simulink library "CockpitDisplayLib"  (R2013b)
settings: Solver=ode45  StartTime=0.0  StopTime=10.0  RelTol=1e-3
undefined symbols (not defined in the file): Ts
libraries: dspadpt3 x3, sf_aircraft_screen_library x1, LandingGearModeLib x1
(part 2 of 2)

== stateflow chart CockpitDisplayLib/Warnings/ComponentModes.RPM ==
  state Normal
    entry: RPMProblem = 0;
  state EngineFailure
    entry:
    RPMProblem = 1;
  state EngineOverSpeed
    entry:
    RPMProblem = 2;
  (default) -> Normal
  Normal -> EngineFailure [order 1] : [funcNormalToEngFailure]
  Normal -> EngineOverSpeed [order 2] : [FlightMode == 1 ...
      | && EngNFuel.RPM >10000]
  EngineFailure -> Normal : [funcEngFailureToNormal]
  EngineOverSpeed -> Normal : [~(FlightMode == 1 ...
      | && EngNFuel.RPM >10000)]
  data: y function_output boolean size=1; y function_output boolean size=1; EngNFuel input Bus: EngineFuel_Bus; RPMProblem output double size=1; FlightMode data_store_memory size=1
  function y = funcEngFailureToNormal:
    | function y = funcEngFailureToNormal
    | 
    | aVarTruthTableCondition_1 = false;
    | aVarTruthTableCondition_2 = false;
    | aVarTruthTableCondition_3 = false;
    | aVarTruthTableCondition_4 = false;
    | 
    | 
    | 
    | aVarTruthTableCondition_1 = logical(FlightMode == 1);
    | 
    | 
    | aVarTruthTableCondition_2 = logical(FlightMode == 2);
    | 
    | 
    | aVarTruthTableCondition_3 = logical(EngNFuel.RPM < 700);
    | 
    | 
    | aVarTruthTableCondition_4 = logical(EngNFuel.RPM < 1500);
    | 
    | if (aVarTruthTableCondition_1 && aVarTruthTableCondition_3)
    |     aFcnTruthTableAction_2();
    | elseif (aVarTruthTableCondition_2 && aVarTruthTableCondition_4)
    |     aFcnTruthTableAction_2();
    | else % Default
    |     aFcnTruthTableAction_1();
    | end
    | 
    | function aFcnTruthTableAction_1()
    | 
    | 
    | y = true;
    | 
    | function aFcnTruthTableAction_2()
    | 
    | 
    | y = false;
  function y = funcNormalToEngFailure:
    | function y = funcNormalToEngFailure
    | 
    | aVarTruthTableCondition_1 = false;
    | aVarTruthTableCondition_2 = false;
    | aVarTruthTableCondition_3 = false;
    | aVarTruthTableCondition_4 = false;
    | 
    | 
    | % Is the aircraft in the PushbackAndTaxi phase
    | 
    | aVarTruthTableCondition_1 = logical(FlightMode == 1);
    | 
    | % Is the aircraft in the TakeoffCruiseDescent phase
    | 
    | aVarTruthTableCondition_2 = logical(FlightMode == 2);
    | 
    | % Lower Threshold for engine speed in PushbackAndTaxi
    | 
    | aVarTruthTableCondition_3 = logical(EngNFuel.RPM < 650);
    | 
    | % Lower Threshold for engine speed in TakeoffCruiseDescent
    | 
    | aVarTruthTableCondition_4 = logical(EngNFuel.RPM < 1500);
    | 
    | if (aVarTruthTableCondition_1 && aVarTruthTableCondition_3)
    |     aFcnTruthTableAction_1();
    | elseif (aVarTruthTableCondition_2 && aVarTruthTableCondition_4)
    |     aFcnTruthTableAction_1();
    | else % Default
    |     aFcnTruthTableAction_2();
    | end
    | 
    | function aFcnTruthTableAction_1()
    | 
    | % The engine speed is lower than the threshold, indicating failure
    | 
    | y = true;
    | 
    | function aFcnTruthTableAction_2()
    | 
    | % The engine speed is above the lower threshold, indicating normal operation
    | 
    | y = false;

== stateflow chart CockpitDisplayLib/Warnings/ComponentModes.Temp ==
  state Normal
    entry: TempProblem = 0;
  state Cooling
  state Heating
  state EngineFire
    entry: TempProblem = 1;
  (default) -> Normal
  Normal -> Heating : [EngNFuel.temperature >2000]
  Heating -> Normal [order 2] : [EngNFuel.temperature <= 2000]
  Cooling -> Normal [order 2] : after(.2,sec)[EngNFuel.temperature <=2000]
  Cooling -> EngineFire [order 1] : [EngNFuel.temperature >2000]
  EngineFire -> Cooling : [EngNFuel.temperature <=2000]
  Heating -> EngineFire [order 1] : after(.2,sec)[EngNFuel.temperature >2000]
  data: EngNFuel input Bus: EngineFuel_Bus; TempProblem output double size=1
